simulink model "lorenz_system"  (R2024b)
settings: Solver=VariableStepAuto  StartTime=0.0  StopTime=100  RelTol=1e-3
settings Model: Creator=Botló  LastModifiedBy=Botló

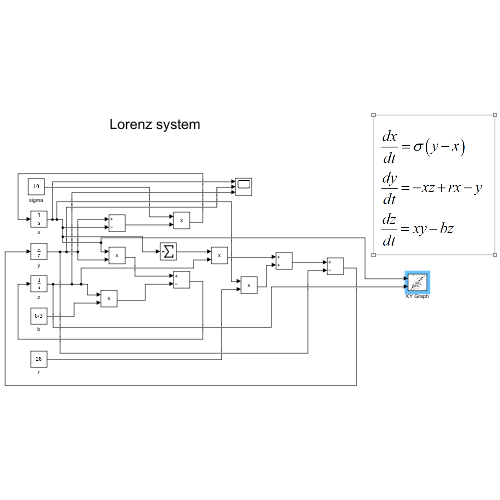
[thumbnail: Simulink's stored preview of the top-level diagram]
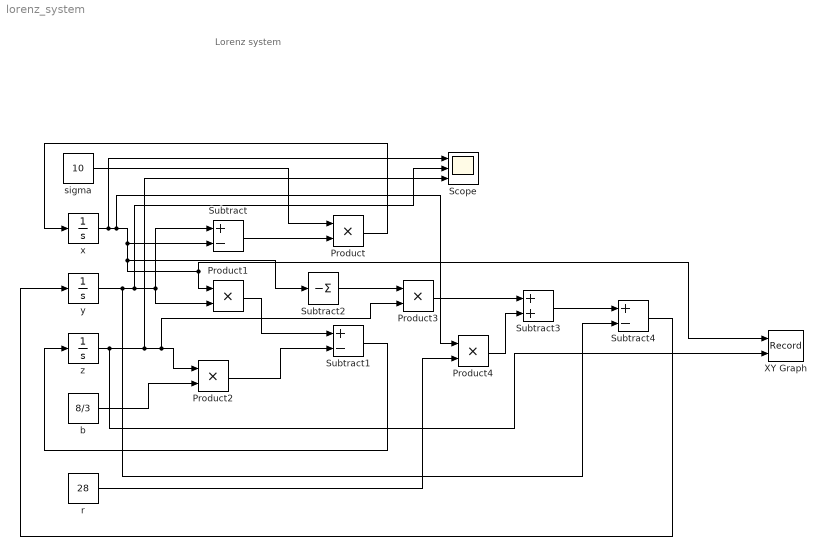
== system lorenz_system ==
  note: Lorenz system
  Product{,1..4} (5 alike) : Product
  Scope : Scope  NumInputPorts=3
  Subtract : Sum  Inputs=+-
  Subtract1 : Sum  Inputs=+-
  Subtract2 : Sum  Inputs=-
  Subtract3 : Sum
  Subtract4 : Sum  Inputs=+-
  XY Graph : Record  FileSettingsInternal="{\"entries\":[{\"content\":{\"excelSettings\":{\"content\":{},\"type\":\"Streamout.ExcelSettings\"}},\"type\":\"Streamout.FileSettingStorage\",\"uuid\":\"\"}],\"packageUris\":[\"http:\\/\\/schema.mathworks.com\\/mf0\\/streamout_blocks\\/R2020a\"],\"version\":\"1.0\"}"  Layout=[1 1]  SignalsInternal="{\"entries\":[{\"content\":{\"signals\":[{\"content\":{\"blockPath\":[],\"dimensions\":[1],\"domain\":\"\",\"lineColor\":\"#a2142f\",\"plots\":[ 1 ],\"port\":1,\"sid\":[\"\"],\"signalID\":1,\"signalName\":\"x\"},\"type\":\"RecordBlkView.Signal\",\"uuid\":\"\"},{\"content\":{\"blockPath\":[],\"dimensions\":[1],\"domain\":\"\",\"lineColor\":\"#139fff\",\"plots\":[ 1 ],\"port\":2,\"sid\":[\"\"],\"signalID\":2,\"signalName\":\"z\"},\"type\":\"RecordBlkView.Signal\",\"uuid\":\"\"}]},\"type\":\"RecordBlkView.InputSignals\",\"uuid\":\"\"}],\"packageUris\":[\"http:\\/\\/schema.mathworks.com\\/mf0\\/streamout_blocks\\/R2020a\"],\"version\":\"1.0\"}"  VisualizationBindings="{\"xyplotplugin\":{\"info\":[{\"series\":[{\"bindingParametersList\":[{\"parameter\":\"X-Axis\",\"signalID\":1,\"signalName\":\"x\"},{\"parameter\":\"Y-Axis\",\"signalID\":2,\"signalName\":\"z\"}],\"seriesID\":0}],\"subplotID\":1}]}}"  CompatibilityTag=XY
  b : Constant  Value=8/3
  r : Constant  Value=28
  sigma : Constant  Value=10
  x : Integrator  InitialCondition=1
  y : Integrator  InitialCondition=1
  z : Integrator  InitialCondition=1
  wires:
  y/1 -> Subtract4/2, Scope/2, Product1/2, Subtract/1
  x/1 -> XY Graph/1, Product1/1, Subtract2/1, Subtract/2, Product4/1, Scope/1
  Subtract/1 -> Product/2
  sigma/1 -> Product/1
  Product/1 -> x/1
  b/1 -> Product2/2
  z/1 -> XY Graph/2, Scope/3, Product3/2, Product2/1
  Product2/1 -> Subtract1/2
  Product1/1 -> Subtract1/1
  Subtract1/1 -> z/1
  Subtract2/1 -> Product3/1
  Product3/1 -> Subtract3/1
  Product4/1 -> Subtract3/2
  r/1 -> Product4/2
  Subtract3/1 -> Subtract4/1
  Subtract4/1 -> y/1
